simulink model "engine_Si"  (R2026a)
settings: Solver=VariableStepAuto  StopTime=10
libraries: fl_lib x16, nesl_utility x16, simulink x2, sdl_lib x2, ee_lib x1
settings Model: Creator=doyeop  LastModifiedBy=doyeop
settings SolverCC: ZeroCrossAlgorithm=Adaptive
settings DebuggingCC: IgnoredZcDiagnostic=none

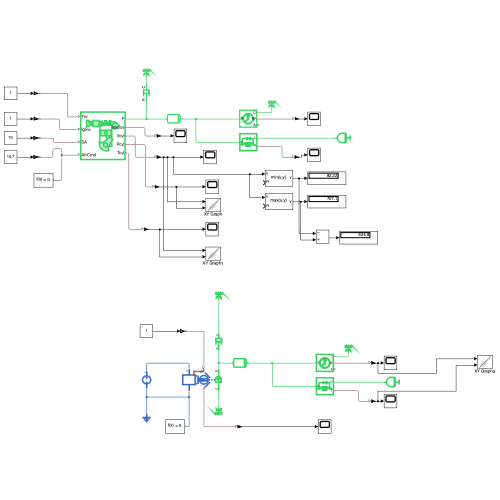
[thumbnail: Simulink's stored preview of the top-level diagram]
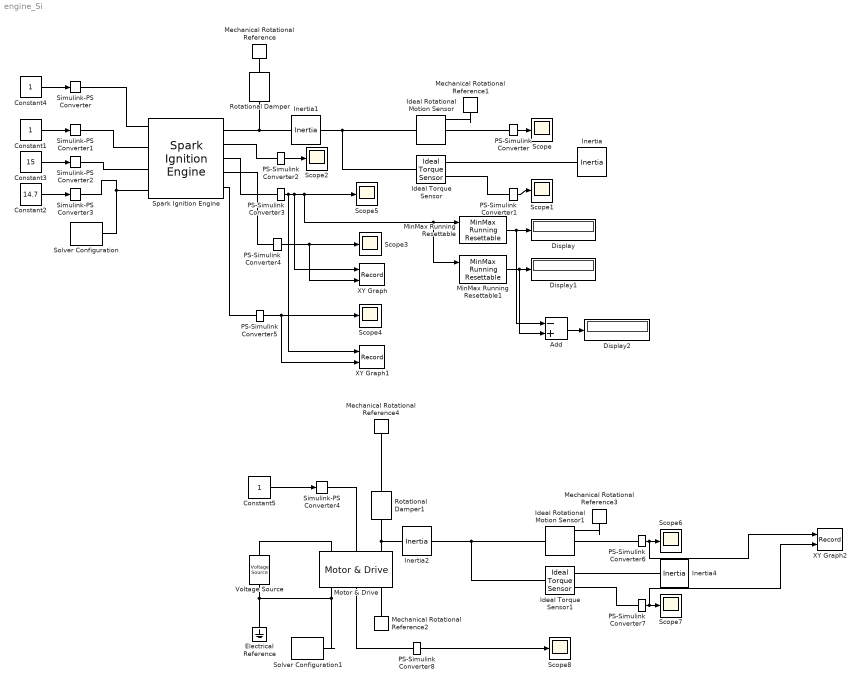
== system engine_Si ==
  Add : Sum  Inputs=-+
  Constant1 : Constant
  Constant2 : Constant  Value=14.7  SampleTime=-1
  Constant3 : Constant  Value=15  SampleTime=-1
  Constant4 : Constant  SampleTime=-1
  Constant5 : Constant  SampleTime=-1
  Display : Display
  Display1 : Display
  Display2 : Display
  Electrical Reference : fl_lib/Electrical/Electrical Elements/Electrical Reference
  Ideal Rotational Motion Sensor : fl_lib/Mechanical/Mechanical Sensors/Ideal Rotational Motion Sensor  reference=foundation.enum.MeasurementReference.difference  acceleration_port=false  velocity_port=true  position_port=true  wrap_angle=false  offset=0 rad
  Ideal Rotational Motion Sensor1 : fl_lib/Mechanical/Mechanical Sensors/Ideal Rotational Motion Sensor  reference=foundation.enum.MeasurementReference.difference  acceleration_port=false  velocity_port=true  position_port=true  wrap_angle=false  offset=0 rad
  Ideal Torque Sensor : fl_lib/Mechanical/Mechanical Sensors/Ideal Torque Sensor
  Ideal Torque Sensor1 : fl_lib/Mechanical/Mechanical Sensors/Ideal Torque Sensor
  Inertia : fl_lib/Mechanical/Rotational Elements/Inertia  inertia=0.1 kg*m^2  num_ports=foundation.enum.numPorts2.one  w_specify=on  w_priority=None  w=0 rpm  w_nominal_specify=off  w_nominal_value=1  w_nominal_unit=rad/s  t_specify=off  t_priority=None  t=0 N*m  t_nominal_specify=off  t_nominal_value=1  t_nominal_unit=N*m
  Inertia1 : fl_lib/Mechanical/Rotational Elements/Inertia  inertia=0.01 kg*m^2  num_ports=foundation.enum.numPorts2.two  w_specify=on  w_priority=High  w=800 rpm  w_nominal_specify=off  w_nominal_value=1  w_nominal_unit=rad/s  t_specify=off  t_priority=None  t=0 N*m  t_nominal_specify=off  t_nominal_value=1  t_nominal_unit=N*m
  Inertia2 : fl_lib/Mechanical/Rotational Elements/Inertia  inertia=0.01 kg*m^2  num_ports=foundation.enum.numPorts2.two  w_specify=on  w_priority=High  w=0 rpm  w_nominal_specify=off  w_nominal_value=1  w_nominal_unit=rad/s  t_specify=off  t_priority=None  t=0 N*m  t_nominal_specify=off  t_nominal_value=1  t_nominal_unit=N*m
  Inertia4 : fl_lib/Mechanical/Rotational Elements/Inertia  inertia=0.1 kg*m^2  num_ports=foundation.enum.numPorts2.one  w_specify=on  w_priority=None  w=0 rpm  w_nominal_specify=off  w_nominal_value=1  w_nominal_unit=rad/s  t_specify=off  t_priority=None  t=0 N*m  t_nominal_specify=off  t_nominal_value=1  t_nominal_unit=N*m
  Mechanical Rotational Reference{,1..4} (5 alike) : fl_lib/Mechanical/Rotational Elements/Mechanical Rotational Reference
  MinMax Running Resettable : simulink/Math Operations/MinMax Running Resettable  Function=min  vinit=inf
  MinMax Running Resettable1 : simulink/Math Operations/MinMax Running Resettable  Function=max  vinit=0.0
  Motor & Drive : sdl_lib/Engines & Motors/Motor & Drive  torque_max=400 N*m  power_max=200 kW  Tc=0.02 s  eff=100  w_eff=3750 rpm  T_eff=100 N*m  thermal_port=simscape.enum.thermaleffects.omit  thermal_mass=100 J/K  temperature_specify=off  temperature_priority=High  temperature=300 K  temperature_nominal_specify=off  temperature_nominal_value=1  temperature_nominal_unit=K
  PS-Simulink Converter : nesl_utility/PS-Simulink Converter  PhysicalDomain=network_engine_domain  SubClassName=ps_output  LeftPortType=input  RightPortType=output  PseudoPeriodic=off  Frequencies=[]  VectorFormat=inherit  Unit=rpm  AffineConversion=off
  PS-Simulink Converter{1..5,7} (6 alike) : nesl_utility/PS-Simulink Converter  PhysicalDomain=network_engine_domain  SubClassName=ps_output  LeftPortType=input  RightPortType=output  PseudoPeriodic=off  Frequencies=[]  VectorFormat=inherit  Unit=inherit  AffineConversion=off
  PS-Simulink Converter6 : nesl_utility/PS-Simulink Converter  PhysicalDomain=network_engine_domain  SubClassName=ps_output  LeftPortType=input  RightPortType=output  PseudoPeriodic=off  Frequencies=[]  VectorFormat=inherit  Unit=rpm  AffineConversion=off
  PS-Simulink Converter8 : nesl_utility/PS-Simulink Converter  PhysicalDomain=network_engine_domain  SubClassName=ps_output  LeftPortType=input  RightPortType=output  PseudoPeriodic=off  Frequencies=[]  VectorFormat=inherit  Unit=rpm  AffineConversion=off
  Rotational Damper : fl_lib/Mechanical/Rotational Elements/Rotational Damper  D=0.01 N*m/rpm  w_specify=off  w_priority=None  w=0 rad/s  w_nominal_specify=off  w_nominal_value=1  w_nominal_unit=rad/s  t_specify=off  t_priority=None  t=0 N*m  t_nominal_specify=off  t_nominal_value=1  t_nominal_unit=N*m
  Rotational Damper1 : fl_lib/Mechanical/Rotational Elements/Rotational Damper  D=0.01 N*m/rpm  w_specify=off  w_priority=None  w=0 rad/s  w_nominal_specify=off  w_nominal_value=1  w_nominal_unit=rad/s  t_specify=off  t_priority=None  t=0 N*m  t_nominal_specify=off  t_nominal_value=1  t_nominal_unit=N*m
  Scope{,1..8} (9 alike) : Scope
      Scope settings: ActiveDisplayYMinimum=273.53511310273376  ActiveDisplayYMaximum=3299.1796535102649
      Scope1 settings: ActiveDisplayYMinimum=-201.61091903355469  ActiveDisplayYMaximum=430.57880541256947
      Scope2 settings: ActiveDisplayYMinimum=-90.0000000000104  ActiveDisplayYMaximum=810.00000000000318  DataLoggingVariableName=ScopeData2
      Scope3 settings: ActiveDisplayYMinimum=-0.15246962816738968  ActiveDisplayYMaximum=2.1728826100903169  DataLoggingVariableName=ScopeData3
      Scope4 settings: ActiveDisplayYMinimum=78.106339439469565  ActiveDisplayYMaximum=2237.8473324158513  DataLoggingVariableName=ScopeData4
      Scope5 settings: ActiveDisplayYMinimum=4.11076155952658  ActiveDisplayYMaximum=785.16664286759  DataLoggingVariableName=ScopeData5
      Scope6 settings: ActiveDisplayYMinimum=-12.497875083356337  ActiveDisplayYMaximum=112.48087575020708  DataLoggingVariableName=ScopeData6
      Scope7 settings: ActiveDisplayYMinimum=4.5691456079700288  ActiveDisplayYMaximum=98.915474260615809  DataLoggingVariableName=ScopeData7
      Scope8 settings: ActiveDisplayYMinimum=-12.497875083356337  ActiveDisplayYMaximum=112.48087575020708  DataLoggingVariableName=ScopeData8
  Simulink-PS Converter{,1,3..4} (4 alike) : nesl_utility/Simulink-PS Converter  PhysicalDomain=network_engine_domain  SubClassName=ps_input  LeftPortType=input  RightPortType=output  PseudoPeriodic=off  Frequencies=[]  NoiseDistribution=none  NoiseParameters=[]  Unit=1  AffineConversion=off  FilteringAndDerivatives=provide  SimscapeFilterOrder=1  InputFilterTimeConstant=0.001  UdotUserProvided=0
  Simulink-PS Converter2 : nesl_utility/Simulink-PS Converter  PhysicalDomain=network_engine_domain  SubClassName=ps_input  LeftPortType=input  RightPortType=output  PseudoPeriodic=off  Frequencies=[]  NoiseDistribution=none  NoiseParameters=[]  Unit=deg  AffineConversion=off  FilteringAndDerivatives=provide  SimscapeFilterOrder=1  InputFilterTimeConstant=0.001  UdotUserProvided=0
  Solver Configuration : nesl_utility/Solver Configuration  PhysicalDomain=network_engine_domain  SubClassName=solver  LeftPortType=input  RightPortType=generic  Tones=[]  Harmonics=[]  SimulateNoise=off  Profile=off  UseLocalSampling=off  EnableSwitchedLinearOptims=on  FrequencyDomain=off  UseCCode=off  RelTol=0.001  AbsTol=0.001  MinStep=1e-09  ToWorkspace=off  RevertToSquareIcSolve=off  NumHomotopyIterations=100  PhasorMode=off  PhasorModeNumHarmonics=1  ConsistencySolver=NEWTON_XTOL_AFTER_FTOL  CanonicalOrdering=CANONICAL  OptimizeIntermediates=OPTIMIZED  IndexReductionMethod=DerivativeReplacement  DoDC=off  ResidualTolerance=1e-09  ConsistencyTolSource=GLOBAL  ConsistencyAbsTol=0.001  ConsistencyRelTol=0.001  ConsistencyTolFactor=0.001  UseLocalSolver=off  LocalSolverChoice=NE_BACKWARD_EULER_ADVANCER  ResolveIndetEquations=on  FunctionEvalNumThread=1  LocalSolverSampleTime=0.001  DoFixedCost=off  MaxNonlinIter=3  MaxModeIter=2  ComputeImpulses=off  ImpulseIterations=2  LinearAlgebra=auto  LinearAlgebraNumThread=0  EquationFormulation=NE_TIME_EF  DelaysMemoryBudget=1024  AutomaticFiltering=on  FilteringTimeConstant=0.001  PartitionStorageMethod=AS_NEEDED  PartitionMemoryBudget=1024  PartitionMethod=ROBUST  MultibodyUseLocalSolver=off  MultibodyLocalSolverChoice=ODE1  MultibodyLocalSolverSampleTime=0.001
  Solver Configuration1 : nesl_utility/Solver Configuration  PhysicalDomain=network_engine_domain  SubClassName=solver  LeftPortType=input  RightPortType=generic  Tones=[]  Harmonics=[]  SimulateNoise=off  Profile=off  UseLocalSampling=off  EnableSwitchedLinearOptims=on  FrequencyDomain=off  UseCCode=off  RelTol=0.001  AbsTol=0.001  MinStep=1e-09  ToWorkspace=off  RevertToSquareIcSolve=off  NumHomotopyIterations=100  PhasorMode=off  PhasorModeNumHarmonics=1  ConsistencySolver=NEWTON_XTOL_AFTER_FTOL  CanonicalOrdering=CANONICAL  OptimizeIntermediates=OPTIMIZED  IndexReductionMethod=DerivativeReplacement  DoDC=off  ResidualTolerance=1e-09  ConsistencyTolSource=GLOBAL  ConsistencyAbsTol=0.001  ConsistencyRelTol=0.001  ConsistencyTolFactor=0.001  UseLocalSolver=off  LocalSolverChoice=NE_BACKWARD_EULER_ADVANCER  ResolveIndetEquations=on  FunctionEvalNumThread=1  LocalSolverSampleTime=0.001  DoFixedCost=off  MaxNonlinIter=3  MaxModeIter=2  ComputeImpulses=off  ImpulseIterations=2  LinearAlgebra=auto  LinearAlgebraNumThread=0  EquationFormulation=NE_TIME_EF  DelaysMemoryBudget=1024  AutomaticFiltering=on  FilteringTimeConstant=0.001  PartitionStorageMethod=AS_NEEDED  PartitionMemoryBudget=1024  PartitionMethod=ROBUST  MultibodyUseLocalSolver=off  MultibodyLocalSolverChoice=ODE1  MultibodyLocalSolverSampleTime=0.001
  Spark Ignition Engine : sdl_lib/Engines & Motors/Spark Ignition Engine  numCyls=sdl.enum.engineNumCylinders.One  twoCylSADiff=270 deg  L4FiringOrder=sdl.enum.engineFiringOrderFourCylinders.L4_1342  bore=91.9 mm  stroke=94.2 mm  conrod=141 mm  CR=8.6  P_amb=101.325 kPa  T_amb=298.15 K  rho_air=1.225 mg/cm^3  R_air=288.1965 J/(K*kg)  UseAirIntake=true  c_thr=0.1 s  thr_rest=3 deg  D_plate=5 cm  S_leak=1 cm^2  V_im=500 cm^3  Cd_in=0.9  IVO_0=-10 deg  IVC_0=100 deg  EVO_0=30 deg  EVC_0=5 deg  UseInVVT=false  UseExVVT=false  q_LHV=44.3 MJ/kg  InputAFR=true  AFR_const=14.6  InputInjPw=false  Sinj=6.5 mg/ms  SparkInputType=sdl.enum.engineSparkInputType.Angle  SA_const=20 deg  comb_bd=50 deg  dt_Pcyl_slow_decay=60 s  dt_Tcyl_slow_decay=600 s  dt_exh_decay=5 ms  InputBackPressure=false  dP_exh=50 kPa  dw_exh=6000 rpm  UseExhaustThermal=true  S_exh=1 m^2  M_exh=5 kg  C_exh=100 J/(K*kg)  k_gas=10 s  h_convection=100 W/(K*m^2)  k_radiation=0.3  SB=5.7e-8 W/(K^4*m^2)  Pim_0=101.325 kPa  ca0=0 deg  w0=800 rpm  EngSpdSimLimit=8500 rpm  OutputTorqueAvr=false  OutputSpeedAvr=false  OutputCrkpos=true  OutputPim=false  OutputAirMassFlow=false  OutputFuelMassFlow=false  OutputAFR=false  OutputVcyl=true  OutputPcyl=true  OutputTcyl=true  OutputTexh=false
  Voltage Source : ee_lib/Sources/Voltage Source  dc_voltage=500 V  ac_voltage=0 V  ac_shift=0 rad  ac_frequency=0 Hz  noise_mode=ee.enum.sources.noise.Disabled  PSD=0 V^2/Hz  sample_time=1e-3 s  repeatability=ee.enum.sources.repeatability.NotRepeatable  user_seed=0  auto_seed=3890346746  i_specify=off  i_priority=None  i=0 A  i_nominal_specify=off  i_nominal_value=1  i_nominal_unit=A  v_specify=off  v_priority=None  v=0 V  v_nominal_specify=off  v_nominal_value=1  v_nominal_unit=V
  XY Graph : Record  NumPorts=2.0  FileSettingsInternal="{\"entries\":[{\"content\":{\"excelSettings\":{\"content\":{},\"type\":\"Streamout.ExcelSettings\"},\"parquetSettings\":{\"content\":{},\"type\":\"Streamout.ParquetSettings\"}},\"type\":\"Streamout.FileSettingStorage\",\"uuid\":\"\"}],\"packageUris\":[\"http:\\/\\/schema.mathworks.com\\/mf0\\/streamout_blocks\\/R2020a\"],\"version\":\"1.0\"}"  FrameSettings=[0, 0]  Layout=[1 1]  SignalsInternal="{\"entries\":[{\"content\":{\"signals\":[{\"content\":{\"blockPath\":[],\"dimensions\":[1],\"domain\":\"\",\"lineColor\":\"#a2142f\",\"plots\":[ 1 ],\"port\":1,\"sid\":[\"\"],\"signalID\":1,\"signalName\":\"PS-Simulink\\nConverter3\"},\"type\":\"RecordBlkView.Signal\",\"uuid\":\"\"},{\"content\":{\"blockPath\":[],\"dimensions\":[1],\"domain\":\"\",\"lineColor\":\"#139fff\",\"plots\":[ 1 ],\"port\":2,\"sid\":[\"\"],\"signalID\":2,\"signalName\":\"PS-Simulink\\nConverter4\"},\"type\":\"RecordBlkView.Signal\",\"uuid\":\"\"}]},\"type\":\"RecordBlkView.InputSignals\",\"uuid\":\"\"}],\"packageUris\":[\"http:\\/\\/schema.mathworks.com\\/mf0\\/streamout_blocks\\/R2020a\"],\"version\":\"1.0\"}"  VisualizationBindings="{\"xyplotplugin\":{\"info\":[{\"series\":[{\"bindingParametersList\":[{\"parameter\":\"X-Axis\",\"signalID\":1,\"signalName\":\"PS-Simulink\\nConverter3\"},{\"parameter\":\"Y-Axis\",\"signalID\":2,\"signalName\":\"PS-Simulink\\nConverter4\"}],\"seriesID\":0}],\"subplotID\":1}]}}"  CompatibilityTag=XY
  XY Graph1 : Record  NumPorts=2.0  FileSettingsInternal="{\"entries\":[{\"content\":{\"excelSettings\":{\"content\":{},\"type\":\"Streamout.ExcelSettings\"},\"parquetSettings\":{\"content\":{},\"type\":\"Streamout.ParquetSettings\"}},\"type\":\"Streamout.FileSettingStorage\",\"uuid\":\"\"}],\"packageUris\":[\"http:\\/\\/schema.mathworks.com\\/mf0\\/streamout_blocks\\/R2020a\"],\"version\":\"1.0\"}"  FrameSettings=[0, 0]  Layout=[1 1]  SignalsInternal="{\"entries\":[{\"content\":{\"signals\":[{\"content\":{\"blockPath\":[],\"dimensions\":[1],\"domain\":\"\",\"lineColor\":\"#a2142f\",\"plots\":[ 1 ],\"port\":1,\"sid\":[\"\"],\"signalID\":1,\"signalName\":\"PS-Simulink\\nConverter3\"},\"type\":\"RecordBlkView.Signal\",\"uuid\":\"\"},{\"content\":{\"blockPath\":[],\"dimensions\":[1],\"domain\":\"\",\"lineColor\":\"#139fff\",\"plots\":[ 1 ],\"port\":2,\"sid\":[\"\"],\"signalID\":2,\"signalName\":\"PS-Simulink\\nConverter5\"},\"type\":\"RecordBlkView.Signal\",\"uuid\":\"\"}]},\"type\":\"RecordBlkView.InputSignals\",\"uuid\":\"\"}],\"packageUris\":[\"http:\\/\\/schema.mathworks.com\\/mf0\\/streamout_blocks\\/R2020a\"],\"version\":\"1.0\"}"  VisualizationBindings="{\"xyplotplugin\":{\"info\":[{\"series\":[{\"bindingParametersList\":[{\"parameter\":\"X-Axis\",\"signalID\":1,\"signalName\":\"PS-Simulink\\nConverter3\"},{\"parameter\":\"Y-Axis\",\"signalID\":2,\"signalName\":\"PS-Simulink\\nConverter5\"}],\"seriesID\":0}],\"subplotID\":1}]}}"  CompatibilityTag=XY
  XY Graph2 : Record  NumPorts=2.0  FileSettingsInternal="{\"entries\":[{\"content\":{\"excelSettings\":{\"content\":{},\"type\":\"Streamout.ExcelSettings\"},\"parquetSettings\":{\"content\":{},\"type\":\"Streamout.ParquetSettings\"}},\"type\":\"Streamout.FileSettingStorage\",\"uuid\":\"\"}],\"packageUris\":[\"http:\\/\\/schema.mathworks.com\\/mf0\\/streamout_blocks\\/R2020a\"],\"version\":\"1.0\"}"  FrameSettings=[0, 0]  Layout=[1 1]  SignalsInternal="{\"entries\":[{\"content\":{\"signals\":[{\"content\":{\"blockPath\":[],\"dimensions\":[1],\"domain\":\"\",\"lineColor\":\"#a2142f\",\"plots\":[ 1 ],\"port\":1,\"sid\":[\"\"],\"signalID\":1,\"signalName\":\"PS-Simulink\\nConverter6\"},\"type\":\"RecordBlkView.Signal\",\"uuid\":\"\"},{\"content\":{\"blockPath\":[],\"dimensions\":[1],\"domain\":\"\",\"lineColor\":\"#139fff\",\"plots\":[ 1 ],\"port\":2,\"sid\":[\"\"],\"signalID\":2,\"signalName\":\"PS-Simulink\\nConverter7\"},\"type\":\"RecordBlkView.Signal\",\"uuid\":\"\"}]},\"type\":\"RecordBlkView.InputSignals\",\"uuid\":\"\"}],\"packageUris\":[\"http:\\/\\/schema.mathworks.com\\/mf0\\/streamout_blocks\\/R2020a\"],\"version\":\"1.0\"}"  VisualizationBindings="{\"xyplotplugin\":{\"info\":[{\"series\":[{\"bindingParametersList\":[{\"parameter\":\"X-Axis\",\"signalID\":1,\"signalName\":\"PS-Simulink\\nConverter6\"},{\"parameter\":\"Y-Axis\",\"signalID\":2,\"signalName\":\"PS-Simulink\\nConverter7\"}],\"seriesID\":0}],\"subplotID\":1}]}}"  CompatibilityTag=XY
  wires:
  Constant4/1 -> Simulink-PS Converter/1
  Constant1/1 -> Simulink-PS Converter1/1
  Constant3/1 -> Simulink-PS Converter2/1
  Constant2/1 -> Simulink-PS Converter3/1
  PS-Simulink Converter/1 -> Scope/1
  PS-Simulink Converter1/1 -> Scope1/1
  PS-Simulink Converter2/1 -> Scope2/1
  PS-Simulink Converter3/1 -> XY Graph1/1, XY Graph/1, MinMax Running Resettable1/1, MinMax Running Resettable/1, Scope5/1
  MinMax Running Resettable/1 -> Add/1, Display/1
  MinMax Running Resettable1/1 -> Add/2, Display1/1
  Add/1 -> Display2/1
  PS-Simulink Converter5/1 -> XY Graph1/2, Scope4/1
  PS-Simulink Converter4/1 -> XY Graph/2, Scope3/1
  PS-Simulink Converter6/1 -> XY Graph2/1, Scope6/1
  PS-Simulink Converter7/1 -> XY Graph2/2, Scope7/1
  Constant5/1 -> Simulink-PS Converter4/1
  PS-Simulink Converter8/1 -> Scope8/1
  connections:
  Simulink-PS Converter/RConn1 -- Spark Ignition Engine/LConn1
  Simulink-PS Converter1/RConn1 -- Spark Ignition Engine/LConn2
  Simulink-PS Converter2/RConn1 -- Spark Ignition Engine/LConn3
  Simulink-PS Converter3/RConn1 -- Solver Configuration/RConn1 -- Spark Ignition Engine/LConn4
  Rotational Damper/LConn1 -- Inertia1/RConn1 -- Spark Ignition Engine/RConn1
  Mechanical Rotational Reference/LConn1 -- Rotational Damper/RConn1
  Ideal Torque Sensor/LConn1 -- Inertia1/LConn1 -- Ideal Rotational Motion Sensor/LConn1
  PS-Simulink Converter/LConn1 -- Ideal Rotational Motion Sensor/RConn2
  Inertia/LConn1 -- Ideal Torque Sensor/RConn1
  PS-Simulink Converter1/LConn1 -- Ideal Torque Sensor/RConn2
  PS-Simulink Converter2/LConn1 -- Spark Ignition Engine/RConn2
  Mechanical Rotational Reference1/LConn1 -- Ideal Rotational Motion Sensor/RConn1
  PS-Simulink Converter3/LConn1 -- Spark Ignition Engine/RConn3
  PS-Simulink Converter4/LConn1 -- Spark Ignition Engine/RConn4
  PS-Simulink Converter5/LConn1 -- Spark Ignition Engine/RConn5
  Voltage Source/LConn1 -- Motor & Drive/LConn1
  Voltage Source/RConn1 -- Electrical Reference/LConn1 -- Solver Configuration1/RConn1 -- Motor & Drive/RConn1
  Mechanical Rotational Reference2/LConn1 -- Motor & Drive/RConn3
  Inertia2/RConn1 -- Rotational Damper1/LConn1 -- Motor & Drive/LConn3
  Ideal Rotational Motion Sensor1/LConn1 -- Inertia2/LConn1 -- Ideal Torque Sensor1/LConn1
  Mechanical Rotational Reference3/LConn1 -- Ideal Rotational Motion Sensor1/RConn1
  Inertia4/LConn1 -- Ideal Torque Sensor1/RConn1
  PS-Simulink Converter7/LConn1 -- Ideal Torque Sensor1/RConn2
  PS-Simulink Converter6/LConn1 -- Ideal Rotational Motion Sensor1/RConn2
  Mechanical Rotational Reference4/LConn1 -- Rotational Damper1/RConn1
  Simulink-PS Converter4/RConn1 -- Motor & Drive/LConn2
  PS-Simulink Converter8/LConn1 -- Motor & Drive/RConn2
